simulink model "Askhsh_1"  (R2018b)
settings: Solver=VariableStepAuto  StartTime=0.0  StopTime=10.0  RelTol=1e-3
settings Model: Creator=Giannis  LastModifiedBy=Giannis
settings DataIOCC: Refine=10

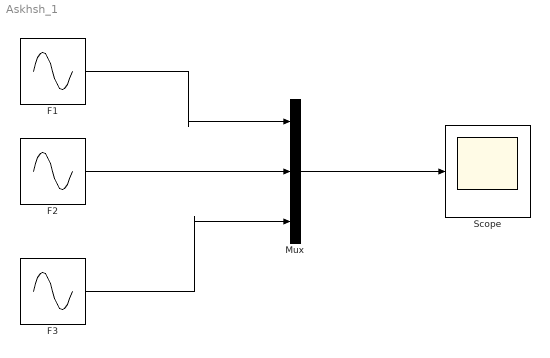
== system Askhsh_1 ==
  F1 : Sin  Amplitude=4  Frequency=pi  SampleTime=0
  F2 : Sin  Amplitude=4  Frequency=pi  Phase=pi/2  SampleTime=0
  F3 : Sin  Amplitude=4  Frequency=pi  Phase=-pi/3  SampleTime=0
  Mux : Mux  Inputs=3
  Scope : Scope
  wires:
  Mux/1 -> Scope/1
  F1/1 -> Mux/1
  F2/1 -> Mux/2
  F3/1 -> Mux/3
